simulink model "PPRZ_act_block_ucorr"  (R2016b)
settings: Solver=VariableStepAuto  StartTime=0.0  StopTime=10.0  RelTol=1e-3
undefined symbols (not defined in the file or in its folder): pars
settings Model: Creator=kkajak  LastModifiedBy=Karl

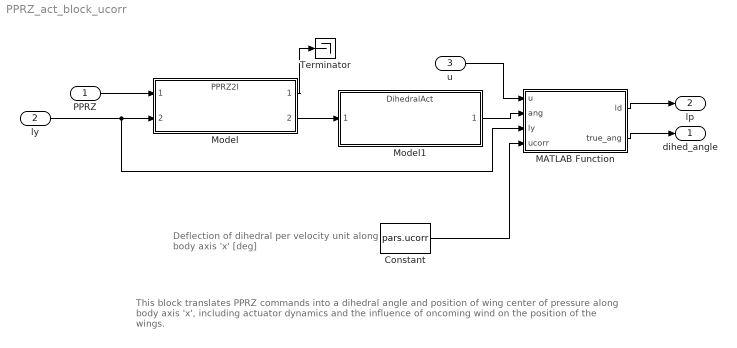
== system PPRZ_act_block_ucorr ==
  note: Deflection of dihedral per velocity unit along
      | body axis 'x' [deg]
  note: This block translates PPRZ commands into a dihedral angle and position of wing center of pressure
      | along body axis 'x', including actuator dynamics and the influence of oncoming wind on the position
      | of the wings.
  PPRZ : Inport
  ly : Inport  Port=2
  u : Inport  Port=3
  Constant : Constant  Value=pars.ucorr
  MATLAB Function : MATLAB Function  TreatAsAtomicUnit=on
  Model : ModelReference  ModelNameDialog=PPRZ2l  SimulationMode=Normal  ModelReferenceVersion=1.7
  Model1 : ModelReference  ModelNameDialog=DihedralAct  SimulationMode=Normal  ModelReferenceVersion=1.2
  Terminator : Terminator
  dihed_angle : Outport
  lp : Outport  Port=2
  wires:
  PPRZ/1 -> Model/1
  ly/1 -> MATLAB Function/3(ly), Model/2
  Model/2 -> Model1/1
  Model/1 -> Terminator/1
  Model1/1 -> MATLAB Function/2(ang)
  u/1 -> MATLAB Function/1(u)
  MATLAB Function/1(ld) -> lp/1
  MATLAB Function/2(true_ang) -> dihed_angle/1
  Constant/1 -> MATLAB Function/4(ucorr)

== matlab function PPRZ_act_block_ucorr/MATLAB Function ==
  data: u input; ld output; ang input; ly input; true_ang output; ucorr input
function [ld,true_ang] = fcn(u,ang,ly,ucorr)

true_ang = (ang + u*ucorr)/180*pi;
ld = ly*sin(true_ang);
